simulink model "miqp_trajectories_visualize"  (R2016b)
settings: Solver=VariableStepAuto  StartTime=0.0  StopTime=10.0  RelTol=1e-3
libraries: vrlib x4
settings Model: Creator=exx  LastModifiedBy=exx

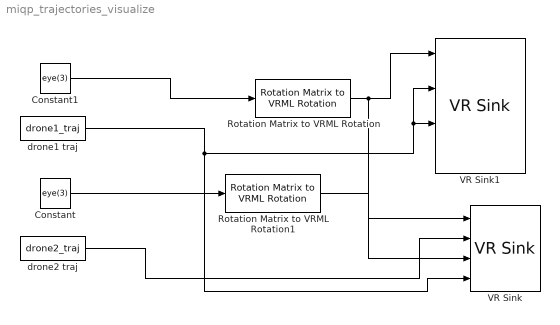
== system miqp_trajectories_visualize ==
  Constant : Constant  Value=eye(3)
  Constant1 : Constant  Value=eye(3)
  Rotation Matrix to VRML Rotation : vrlib/Utilities/Rotation Matrix to VRML Rotation  maxzero=1e-12
  Rotation Matrix to VRML Rotation1 : vrlib/Utilities/Rotation Matrix to VRML Rotation  maxzero=1e-12
  VR Sink : vrlib/VR Sink  InstantiateOnLoad=on  SampleTime=0.1  ViewEnable=on  RemoteChange=off  RemoteView=off  FieldsWritten=copter2.rotation.4.1.1.double#copter2.translation.3.1.1.double#copter.rotation.4.1.1.double#copter.translation.3.1.1.double  WorldFileName=multicopter_world.wrl  AutoView=off  VideoDimensions=[]  AllowVariableSize=off
  VR Sink1 : vrlib/VR Sink  InstantiateOnLoad=on  SampleTime=0.1  ViewEnable=on  RemoteChange=off  RemoteView=off  FieldsWritten=copter.rotation.4.1.1.double#copter.translation.3.1.1.double#vp.translation.3.1.1.double#target.translation.3.1.1.double  WorldFileName=copter_world_wtarget.wrl  AutoView=off  VideoDimensions=[]  AllowVariableSize=off
  drone1 traj : FromWorkspace  VariableName=drone1_traj  SampleTime=0
  drone2 traj : FromWorkspace  VariableName=drone2_traj  SampleTime=0
  wires:
  Rotation Matrix to VRML Rotation/1 -> VR Sink/3, VR Sink1/1
  Constant1/1 -> Rotation Matrix to VRML Rotation/1
  Constant/1 -> Rotation Matrix to VRML Rotation1/1
  Rotation Matrix to VRML Rotation1/1 -> VR Sink/1
  drone1 traj/1 -> VR Sink/4, VR Sink1/3, VR Sink1/2
  drone2 traj/1 -> VR Sink/2
